simulink model "IFAC20_Random_Exp1_C1"  (R2019a)
settings: Solver=ode45  StartTime=0.0  StopTime=60  FixedStep=0.05  MaxStep=0.06  RelTol=1e-3  EnableMultiTasking=on
model workspace (MAT data in the model file):
  MCOS : class17 (value not decoded)
values from neighbouring files (symbols this model uses):
  motor_trigger = 1.1    [IFAC20_Experiment2.m]    (also in IFAC20_Experiment3.m = 0.9; IFAC20_Experiment4.m = 0.9)
  wind_trigger = 0.9    [IFAC20_Experiment2.m]    (also in IFAC20_Experiment3.m; IFAC20_Experiment4.m)
undefined symbols (not defined in the file or in its folder): altitude_error, Continuous, IC, quadModel, RPM1, RPM2, RPM3, RPM4, Time
libraries: simulink x10, ctrlSharedLib x4
(part 2 of 2)

== system IFAC20_Random_Exp1_C1/Quadcopter Dynamics/Motor Dynamics/Subsystem ==
  note: kalman filter
  note: Multiplicitive Fault
  In1 : Inport
  In2 : Inport  Port=2
  Kalman Filter : ctrlSharedLib/Kalman Filter  TimeDomain=Continuous-Time  UseCurrentEstimator=on  ModelSource=Individual A, B, C, D matrices  ModelSourceVariable=quadcopterDynamicsSFunction  A=-1/quadModel.T  B=1  C=1/quadModel.T  D=0  NumberOfStates=1  NumberOfInputs=1  NumberOfOutputs=1  InitialEstimateSource=Dialog  X0=0  P0=10  UseK=off  UseGH=off  NumberOfProcessNoiseInputs=1  G=1  TimeInvariantG=on  H=0  TimeInvariantH=on  Q=0.05  TimeInvariantQ=on  R=1  TimeInvariantR=on  N=0  TimeInvariantN=on  AddInputPort=on  AddEnablePort=off  OutputEstimatedY=on  OutputP=off  Ts=-1
      settings: SourceProductBaseCode=CT
  MATLAB Function : MATLAB Function  TreatAsAtomicUnit=on
  Motor_Dynamics_1 : StateSpace  A=-1/quadModel.T  C=1/quadModel.T  D=0  InitialCondition=IC.w1*quadModel.T
  Out1 : Outport
  Out2 : Outport  Port=2
  wires:
  In1/1 -> Kalman Filter/1, Motor_Dynamics_1/1
  MATLAB Function/1(rotor_speed) -> Out1/1, Kalman Filter/2
  In2/1 -> MATLAB Function/1(fault)
  Motor_Dynamics_1/1 -> MATLAB Function/2(nominal_model_input)
  Kalman Filter/2 -> Out2/1

== system IFAC20_Random_Exp1_C1/Quadcopter Dynamics/Motor Dynamics/Subsystem1 ==
  In1 : Inport
  In2 : Inport  Port=2
  Kalman Filter : ctrlSharedLib/Kalman Filter  TimeDomain=Continuous-Time  UseCurrentEstimator=on  ModelSource=Individual A, B, C, D matrices  ModelSourceVariable=quadcopterDynamicsSFunction  A=-1/quadModel.T  B=1  C=1/quadModel.T  D=0  NumberOfStates=1  NumberOfInputs=1  NumberOfOutputs=1  InitialEstimateSource=Dialog  X0=0  P0=10  UseK=off  UseGH=off  NumberOfProcessNoiseInputs=1  G=1  TimeInvariantG=on  H=0  TimeInvariantH=on  Q=0.05  TimeInvariantQ=on  R=1  TimeInvariantR=on  N=0  TimeInvariantN=on  AddInputPort=on  AddEnablePort=off  OutputEstimatedY=on  OutputP=off  Ts=-1
      settings: SourceProductBaseCode=CT
  MATLAB Function : MATLAB Function  TreatAsAtomicUnit=on
  "Motor_Dynamics_2 " : StateSpace  A=-1/quadModel.T  C=1/quadModel.T  D=0  InitialCondition=IC.w1*quadModel.T
  Out1 : Outport
  Out2 : Outport  Port=2
  wires:
  In1/1 -> "Motor_Dynamics_2 "/1, Kalman Filter/1
  MATLAB Function/1(rotor_speed) -> Kalman Filter/2, Out1/1
  In2/1 -> MATLAB Function/1(fault)
  "Motor_Dynamics_2 "/1 -> MATLAB Function/2(nominal_modal_input)
  Kalman Filter/2 -> Out2/1

== system IFAC20_Random_Exp1_C1/Quadcopter Dynamics/Motor Dynamics/Subsystem2 ==
  In1 : Inport
  In2 : Inport  Port=2
  Kalman Filter : ctrlSharedLib/Kalman Filter  TimeDomain=Continuous-Time  UseCurrentEstimator=on  ModelSource=Individual A, B, C, D matrices  ModelSourceVariable=quadcopterDynamicsSFunction  A=-1/quadModel.T  B=1  C=1/quadModel.T  D=0  NumberOfStates=1  NumberOfInputs=1  NumberOfOutputs=1  InitialEstimateSource=Dialog  X0=0  P0=10  UseK=off  UseGH=off  NumberOfProcessNoiseInputs=1  G=1  TimeInvariantG=on  H=0  TimeInvariantH=on  Q=0.05  TimeInvariantQ=on  R=1  TimeInvariantR=on  N=0  TimeInvariantN=on  AddInputPort=on  AddEnablePort=off  OutputEstimatedY=on  OutputP=off  Ts=-1
      settings: SourceProductBaseCode=CT
  MATLAB Function : MATLAB Function  TreatAsAtomicUnit=on
  "Motor_Dynamics_3 " : StateSpace  A=-1/quadModel.T  C=1/quadModel.T  D=0  InitialCondition=IC.w1*quadModel.T
  Out1 : Outport
  Out2 : Outport  Port=2
  wires:
  In1/1 -> "Motor_Dynamics_3 "/1, Kalman Filter/1
  MATLAB Function/1(rotor_speed) -> Kalman Filter/2, Out1/1
  In2/1 -> MATLAB Function/1(fault)
  "Motor_Dynamics_3 "/1 -> MATLAB Function/2(nominal_modal_input)
  Kalman Filter/2 -> Out2/1

== system IFAC20_Random_Exp1_C1/Quadcopter Dynamics/Motor Dynamics/Subsystem3 ==
  In1 : Inport
  In2 : Inport  Port=2
  Kalman Filter : ctrlSharedLib/Kalman Filter  TimeDomain=Continuous-Time  UseCurrentEstimator=on  ModelSource=Individual A, B, C, D matrices  ModelSourceVariable=quadcopterDynamicsSFunction  A=-1/quadModel.T  B=1  C=1/quadModel.T  D=0  NumberOfStates=1  NumberOfInputs=1  NumberOfOutputs=1  InitialEstimateSource=Dialog  X0=0  P0=10  UseK=off  UseGH=off  NumberOfProcessNoiseInputs=1  G=1  TimeInvariantG=on  H=0  TimeInvariantH=on  Q=0.05  TimeInvariantQ=on  R=1  TimeInvariantR=on  N=0  TimeInvariantN=on  AddInputPort=on  AddEnablePort=off  OutputEstimatedY=on  OutputP=off  Ts=-1
      settings: SourceProductBaseCode=CT
  MATLAB Function : MATLAB Function  TreatAsAtomicUnit=on
  "Motor_Dynamics_4 " : StateSpace  A=-1/quadModel.T  C=1/quadModel.T  D=0  InitialCondition=IC.w1*quadModel.T
  Out1 : Outport
  Out2 : Outport  Port=2
  wires:
  In1/1 -> Kalman Filter/1, "Motor_Dynamics_4 "/1
  MATLAB Function/1(rotor_speed) -> Kalman Filter/2, Out1/1
  In2/1 -> MATLAB Function/1(fault)
  "Motor_Dynamics_4 "/1 -> MATLAB Function/2(nominal_modal_input)
  Kalman Filter/2 -> Out2/1

== system IFAC20_Random_Exp1_C1/Quadcopter Dynamics/Motor Dynamics/Throttle To RPM Gain and Cutoff_1 ==
  note: minThr should be a quad.mat value
  note: This gain should be a quad.mat value
  note: This constant should be a quad.mat value
  note: Output equals linearly scaled RPM
      | for given throttle input if throttle input >=Throttle Cuttoff (minThr)
      | else output is zero.
  In5 : Inport
  Constant : Constant  Value=quadModel.b
  Gain : Gain  Gain=quadModel.cr
  Minimum Throttle Cutoff : simulink/Logic and Bit Operations/Compare To Constant  relop=>=  const=quadModel.minThr  OutDataTypeStr=uint8
  Product : Product
  Sum1 : Sum  Inputs=++|
  Out5 : Outport
  wires:
  Minimum Throttle Cutoff/1 -> Product/2
  Product/1 -> Out5/1
  In5/1 -> Gain/1, Minimum Throttle Cutoff/1
  Gain/1 -> Sum1/2
  Sum1/1 -> Product/1
  Constant/1 -> Sum1/1

== system IFAC20_Random_Exp1_C1/Quadcopter Dynamics/Motor Dynamics/Throttle To RPM Gain and Cutoff_2 ==
  note: minThr should be a quad.mat value
  note: This gain should be a quad.mat value
  note: This constant should be a quad.mat value
  note: Output equals linearly scaled RPM
      | for given throttle input if throttle input >=Throttle Cuttoff (minThr)
      | else output is zero.
  In5 : Inport
  Constant : Constant  Value=quadModel.b
  Gain : Gain  Gain=quadModel.cr
  Minimum Throttle Cutoff : simulink/Logic and Bit Operations/Compare To Constant  relop=>=  const=quadModel.minThr  OutDataTypeStr=uint8
  Product : Product
  Sum1 : Sum  Inputs=++|
  Out5 : Outport
  wires:
  Minimum Throttle Cutoff/1 -> Product/2
  Product/1 -> Out5/1
  In5/1 -> Gain/1, Minimum Throttle Cutoff/1
  Gain/1 -> Sum1/2
  Sum1/1 -> Product/1
  Constant/1 -> Sum1/1

== system IFAC20_Random_Exp1_C1/Quadcopter Dynamics/Motor Dynamics/Throttle To RPM Gain and Cutoff_3 ==
  note: minThr should be a quad.mat value
  note: This gain should be a quad.mat value
  note: This constant should be a quad.mat value
  note: Output equals linearly scaled RPM
      | for given throttle input if throttle input >=Throttle Cuttoff (minThr)
      | else output is zero.
  In5 : Inport
  Constant : Constant  Value=quadModel.b
  Gain : Gain  Gain=quadModel.cr
  Minimum Throttle Cutoff : simulink/Logic and Bit Operations/Compare To Constant  relop=>=  const=quadModel.minThr  OutDataTypeStr=uint8
  Product : Product
  Sum1 : Sum  Inputs=++|
  Out5 : Outport
  wires:
  Minimum Throttle Cutoff/1 -> Product/2
  Product/1 -> Out5/1
  In5/1 -> Gain/1, Minimum Throttle Cutoff/1
  Gain/1 -> Sum1/2
  Sum1/1 -> Product/1
  Constant/1 -> Sum1/1

== system IFAC20_Random_Exp1_C1/Quadcopter Dynamics/Motor Dynamics/Throttle To RPM Gain and Cutoff_4 ==
  note: minThr should be a quad.mat value
  note: This gain should be a quad.mat value
  note: This constant should be a quad.mat value
  note: Output equals linearly scaled RPM
      | for given throttle input if throttle input >=Throttle Cuttoff (minThr)
      | else output is zero.
  In5 : Inport
  Constant : Constant  Value=quadModel.b
  Gain : Gain  Gain=quadModel.cr
  Minimum Throttle Cutoff : simulink/Logic and Bit Operations/Compare To Constant  relop=>=  const=quadModel.minThr  OutDataTypeStr=uint8
  Product : Product
  Sum1 : Sum  Inputs=++|
  Out5 : Outport
  wires:
  Minimum Throttle Cutoff/1 -> Product/2
  Product/1 -> Out5/1
  In5/1 -> Gain/1, Minimum Throttle Cutoff/1
  Gain/1 -> Sum1/2
  Sum1/1 -> Product/1
  Constant/1 -> Sum1/1

== matlab function IFAC20_Random_Exp1_C1/Quadcopter Dynamics/Motor Dynamics/Subsystem/MATLAB Function ==
  data: fault input; nominal_model_input input; rotor_speed output
function rotor_speed = fcn(fault, nominal_model_input)

rotor_speed =(nominal_model_input* (1-fault));

end

== matlab function IFAC20_Random_Exp1_C1/Attitude Controller/blending  ==
  settings: updateMethod=DISCRETE
  data: control_signal output; nominal_controller input
function control_signal  = blending(nominal_controller)


control_signal = nominal_controller;

end

== matlab function IFAC20_Random_Exp1_C1/Quadcopter Dynamics/Motor Dynamics/Subsystem1/MATLAB Function ==
  data: fault input; nominal_modal_input input; rotor_speed output
function rotor_speed = fcn(  fault, nominal_modal_input)


rotor_speed =  (nominal_modal_input* (1-fault));

end

== matlab function IFAC20_Random_Exp1_C1/Position Controller/MATLAB Function ==
  settings: updateMethod=DISCRETE
  data: y_error input; x_error input; max_error_signal data_store_memory; count data_store_memory; time input; prevTime data_store_memory
function fcn(y_error,x_error,time)
global prevTime;
global max_error_signal;
global count;
%if(abs(y_error) + abs(x_error) > max_error_signal)
if(prevTime+0.1 < time)
    max_error_signal = max_error_signal + abs(y_error) + abs(x_error);
    count =count +1;
    %disp(count);
    prevTime = time;
end
end

== matlab function IFAC20_Random_Exp1_C1/Quadcopter Dynamics/Motor Dynamics/Subsystem2/MATLAB Function ==
  data: fault input; nominal_modal_input input; rotor_speed output
function rotor_speed = fcn(  fault, nominal_modal_input)


rotor_speed =  (nominal_modal_input* (1-fault));

end

== matlab function IFAC20_Random_Exp1_C1/Quadcopter Dynamics/Motor Dynamics/Subsystem3/MATLAB Function ==
  data: fault input; nominal_modal_input input; rotor_speed output
function rotor_speed = fcn(  fault, nominal_modal_input)


rotor_speed =  (nominal_modal_input* (1-fault));

end

== matlab function IFAC20_Random_Exp1_C1/Attitude Controller/blending 1 ==
  settings: updateMethod=DISCRETE
  data: control_signal output; nominal_controller input
function control_signal   = blending(nominal_controller)

control_signal =  nominal_controller;

end

== matlab function IFAC20_Random_Exp1_C1/Attitude Controller/blending 2 ==
  data: control_signal output; portion input; fault_controller input; nominal_controller input
function control_signal = blending(portion , fault_controller, nominal_controller)

fault_part = (fault_controller * portion);
nominal_portion = 1-portion;
nominal_part = nominal_controller * nominal_portion;
control_signal = fault_part + nominal_part;

end

== matlab function IFAC20_Random_Exp1_C1/Quadcopter Dynamics/External Disturbances1/MATLAB Function2 ==
  data: mag input; f1 output; switch_signal input; f2 output; f3 output
function [f1,f2,f3] = fcn(mag , switch_signal)

f1 = 0;
f2 = 0;
f3 = 0;

if switch_signal == 1
    f1 = mag;
elseif switch_signal ==2
    f2 = mag;
elseif switch_signal ==3
    f3 = mag;
end

== matlab function IFAC20_Random_Exp1_C1/Position Controller/MATLAB Function1 ==
  settings: updateMethod=DISCRETE
  data: alt_diff input; y output; altitude_error data_store_memory; time input; PrevTime2 data_store_memory
function y = fcn(alt_diff, time)
global altitude_error;
global PrevTime2;

if(PrevTime2+0.1 < time)
    altitude_error = altitude_error + abs(alt_diff);

    y = altitude_error;
    PrevTime2 = time;
else
    y = altitude_error;
end

== matlab function IFAC20_Random_Exp1_C1/Quadcopter Dynamics/Motor Dynamics/MATLAB Function ==
  settings: updateMethod=DISCRETE
  data: oneRes input; twoRes input; threeRes input; fourRes input; fault_est data_store_memory
function fcn(oneRes, twoRes, threeRes, fourRes)
global fault_est;
maxRes = max([oneRes twoRes threeRes fourRes]);
%threshold in rpm
threshold = 50;

if(maxRes > threshold)
    fault_est = 1;
else
    fault_est = 0;
end

== matlab function IFAC20_Random_Exp1_C1/Position Controller/Position Randomization ==
  settings: updateMethod=DISCRETE
  data: Xd input; Xr input; Phi output; Theta output; Yd input; Yr input
function [Phi, Theta] = fcn(Xd, Xr, Yd, Yr)

pos = [Xd, Xr, Yd, Yr];
current_error = pdist(pos,'euclidean');
disp(current_error);
random = false;
if( random)
    
    blend = rand();
    %blend =0;
    Phi = blend;
    Theta= blend;
else
    %blend = rand();
    blend =0;
    Phi = blend;
    Theta= blend;
end

== matlab function IFAC20_Random_Exp1_C1/Position Controller/blending 1 ==
  data: Phi_cmd output; portion input; fault_controller input; nominal_controller input
function Phi_cmd = blending(portion , fault_controller, nominal_controller)

fault_part = (fault_controller * portion);
nominal_portion = 1-portion;
nominal_part = nominal_controller * nominal_portion;
Phi_cmd = fault_part + nominal_part;

end

== matlab function IFAC20_Random_Exp1_C1/Position Controller/blending 2 ==
  data: The_cmd output; portion input; fault_controller input; nominal_controller input
function The_cmd = blending(portion , fault_controller, nominal_controller)

fault_part = (fault_controller * portion);
nominal_portion = 1-portion;
nominal_part = nominal_controller * nominal_portion;
The_cmd = fault_part + nominal_part;

end

== matlab function IFAC20_Random_Exp1_C1/Quadcopter Dynamics/External Disturbances1/Random Wind Generator1 ==
  settings: updateMethod=DISCRETE
  data: fault_mag output; rotor output; trigger input; data input; rotor_select input
function [fault_mag,rotor] = fcn( trigger, data, rotor_select)


if(trigger == 1)
    
    fault_mag = data;
    rotor = round(rotor_select);
else
    fault_mag = 0;
    rotor = 0;
end

== matlab function IFAC20_Random_Exp1_C1/Quadcopter Dynamics/Motor Dynamics/MATLAB Function2 ==
  data: mag input; f1 output; switch_signal input; f2 output; f3 output; f4 output
function [f1,f2,f3,f4] = fcn(mag , switch_signal)

f1 = 0;
f2 = 0;
f3 = 0;
f4 = 0;

if switch_signal == 1
    f1 = mag;
elseif switch_signal ==2
    f2 = mag;
elseif switch_signal ==3
    f3 = mag;
elseif switch_signal ==4
    f4 = mag;
end

== matlab function IFAC20_Random_Exp1_C1/Quadcopter Dynamics/Motor Dynamics/Random Wind Generator1 ==
  settings: updateMethod=DISCRETE
  data: fault_mag output; rotor output; trigger input; data input; rotor_select input
function [fault_mag,rotor] = fcn( trigger, data, rotor_select)


    if(trigger == 1)

        fault_mag = data;
        rotor = round(rotor_select);
        
        
    else
        fault_mag = 0;
        rotor = 0;
    end
